simulink model "ee464_hw1_kaantutek_ESR"  (R2022a)
settings: Solver=VariableStepAuto  StartTime=0.0  StopTime=0.5  RelTol=1e-3
libraries: spsGroundLib x14, spsSeriesRLCBranchLib x13, spsCurrentMeasurementLib x7, spsVoltageMeasurementLib x5, spsDCVoltageSourceLib x3, spsDiodeLib x3, spsMosfetLib x3, spsIdealSwitchLib x1, spspowerguiLib x1
settings Model: Creator=mluser  LastModifiedBy=mluser

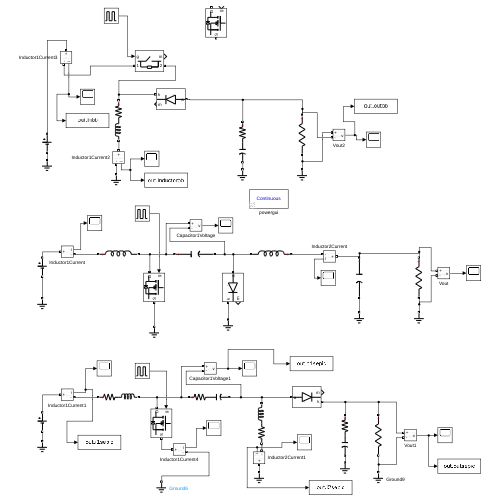
[thumbnail: Simulink's stored preview of the top-level diagram]
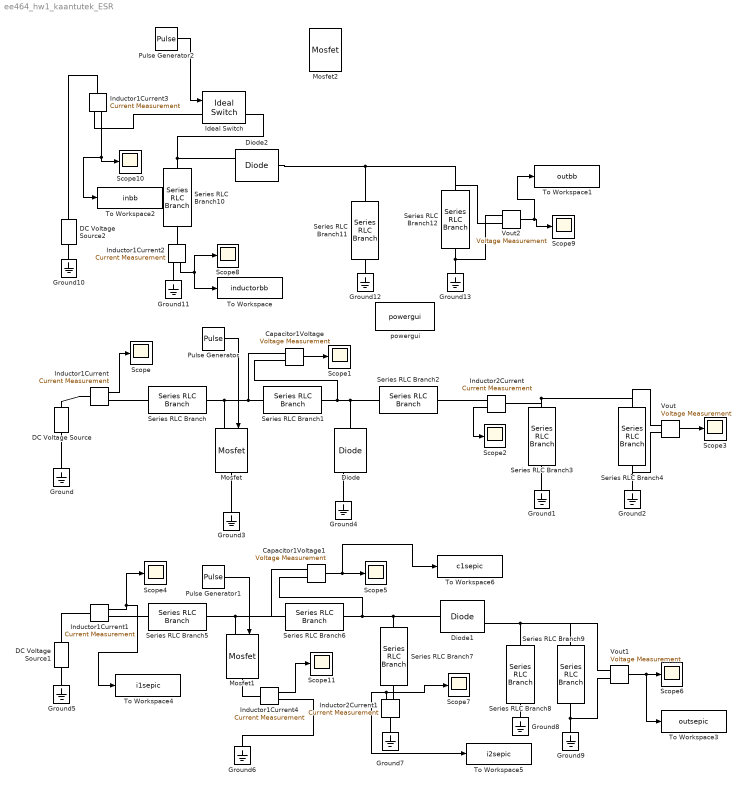
== system ee464_hw1_kaantutek_ESR ==
  Capacitor1Voltage : spsVoltageMeasurementLib/Voltage Measurement  PhasorSimulation=off  OutputType=Complex  PSBequivalent=0
  Capacitor1Voltage1 : spsVoltageMeasurementLib/Voltage Measurement  PhasorSimulation=off  OutputType=Complex  PSBequivalent=0
  DC Voltage Source : spsDCVoltageSourceLib/DC Voltage Source  Amplitude=16  Measurements=None
  DC Voltage Source1 : spsDCVoltageSourceLib/DC Voltage Source  Amplitude=16  Measurements=None
  DC Voltage Source2 : spsDCVoltageSourceLib/DC Voltage Source  Amplitude=16  Measurements=None
  Diode : spsDiodeLib/Diode  Ron=1e-3  Lon=0  Vf=0  IC=0  UseSnubber=0  Rs=0  Cs=0  Measurements=on
  Diode1 : spsDiodeLib/Diode  Ron=1e-3  Lon=0  Vf=0  IC=0  UseSnubber=0  Rs=0  Cs=0  Measurements=on
  Diode2 : spsDiodeLib/Diode  Ron=1e-3  Lon=0  Vf=0  IC=0  UseSnubber=0  Rs=0  Cs=0  Measurements=on
  Ground{,1..13} (14 alike) : spsGroundLib/Ground  LConnTagsString=a
  Ideal Switch : spsIdealSwitchLib/Ideal Switch  Ron=0.001  Lon=0  IC=0  Rs=1e5  Cs=inf  Measurements=on
  Inductor1Current{,1..4} (5 alike) : spsCurrentMeasurementLib/Current Measurement  PhasorSimulation=off  OutputType=Complex  PSBequivalent=0
  Inductor2Current : spsCurrentMeasurementLib/Current Measurement  PhasorSimulation=off  OutputType=Complex  PSBequivalent=0
  Inductor2Current1 : spsCurrentMeasurementLib/Current Measurement  PhasorSimulation=off  OutputType=Complex  PSBequivalent=0
  Mosfet : spsMosfetLib/Mosfet  Ron=1e-6  Lon=0  Rd=1e-6  Vfd=0  IC=0  Rs=1e9  Cs=inf  Measurements=off
  Mosfet1 : spsMosfetLib/Mosfet  Ron=1e-6  Lon=0  Rd=1e-6  Vfd=0  IC=0  Rs=1e9  Cs=inf  Measurements=off
  Mosfet2 : spsMosfetLib/Mosfet  Ron=1e-6  Lon=0  Rd=1e-6  Vfd=0  IC=0  Rs=1e9  Cs=inf  Measurements=off
  Pulse Generator : DiscretePulseGenerator  PulseType=Time based  Amplitude=5  Period=2e-5  PulseWidth=42.857
  Pulse Generator1 : DiscretePulseGenerator  PulseType=Time based  Amplitude=5  Period=2e-5  PulseWidth=42.857
  Pulse Generator2 : DiscretePulseGenerator  PulseType=Time based  Amplitude=5  Period=2e-5  PulseWidth=42.857
  Scope{,1..11} (12 alike) : Scope
  Series RLC Branch : spsSeriesRLCBranchLib/Series RLC Branch  LConnTagsString=__new0  RConnTagsString=__new0  BranchType=L  Resistance=1  Inductance=0.914e-3  SetiL0=off  InitialCurrent=0  Capacitance=1e-6  Setx0=off  InitialVoltage=0  Measurements=None
  Series RLC Branch1 : spsSeriesRLCBranchLib/Series RLC Branch  LConnTagsString=__new0  RConnTagsString=__new0  BranchType=C  Resistance=1  Inductance=1e-3  SetiL0=off  InitialCurrent=0  Capacitance=12.45e-6  Setx0=off  InitialVoltage=0  Measurements=None
  Series RLC Branch10 : spsSeriesRLCBranchLib/Series RLC Branch  LConnTagsString=__new0  RConnTagsString=__new0  BranchType=RL  Resistance=0.048  Inductance=0.470e-3  SetiL0=off  InitialCurrent=0  Capacitance=1e-6  Setx0=off  InitialVoltage=0  Measurements=None
  Series RLC Branch11 : spsSeriesRLCBranchLib/Series RLC Branch  LConnTagsString=__new0  RConnTagsString=__new0  BranchType=RC  Resistance=0.0031  Inductance=1e-3  SetiL0=off  InitialCurrent=0  Capacitance=75e-6  Setx0=off  InitialVoltage=0  Measurements=None
  Series RLC Branch12 : spsSeriesRLCBranchLib/Series RLC Branch  LConnTagsString=__new0  RConnTagsString=__new0  BranchType=R  Resistance=6  Inductance=0  SetiL0=off  InitialCurrent=0  Capacitance=0  Setx0=off  InitialVoltage=0  Measurements=None
  Series RLC Branch2 : spsSeriesRLCBranchLib/Series RLC Branch  LConnTagsString=__new0  RConnTagsString=__new0  BranchType=L  Resistance=1  Inductance=0.686e-3  SetiL0=off  InitialCurrent=0  Capacitance=1e-6  Setx0=off  InitialVoltage=0  Measurements=None
  Series RLC Branch3 : spsSeriesRLCBranchLib/Series RLC Branch  LConnTagsString=__new0  RConnTagsString=__new0  BranchType=C  Resistance=1  Inductance=1e-3  SetiL0=off  InitialCurrent=0  Capacitance=6.12e-6  Setx0=off  InitialVoltage=0  Measurements=None
  Series RLC Branch4 : spsSeriesRLCBranchLib/Series RLC Branch  LConnTagsString=__new0  RConnTagsString=__new0  BranchType=R  Resistance=6  Inductance=0  SetiL0=off  InitialCurrent=0  Capacitance=0  Setx0=off  InitialVoltage=0  Measurements=None
  Series RLC Branch5 : spsSeriesRLCBranchLib/Series RLC Branch  LConnTagsString=__new0  RConnTagsString=__new0  BranchType=RL  Resistance=2.44  Inductance=0.960e-3  SetiL0=off  InitialCurrent=0  Capacitance=1e-6  Setx0=off  InitialVoltage=0  Measurements=None
  Series RLC Branch6 : spsSeriesRLCBranchLib/Series RLC Branch  LConnTagsString=__new0  RConnTagsString=__new0  BranchType=RC  Resistance=10.6e-3  Inductance=1e-3  SetiL0=off  InitialCurrent=0  Capacitance=11e-6  Setx0=off  InitialVoltage=0  Measurements=None
  Series RLC Branch7 : spsSeriesRLCBranchLib/Series RLC Branch  LConnTagsString=__new0  RConnTagsString=__new0  BranchType=RL  Resistance=1.6  Inductance=0.68e-3  SetiL0=off  InitialCurrent=0  Capacitance=1e-6  Setx0=off  InitialVoltage=0  Measurements=None
  Series RLC Branch8 : spsSeriesRLCBranchLib/Series RLC Branch  LConnTagsString=__new0  RConnTagsString=__new0  BranchType=RC  Resistance=5.2e-3  Inductance=1e-3  SetiL0=off  InitialCurrent=0  Capacitance=95e-6  Setx0=off  InitialVoltage=0  Measurements=None
  Series RLC Branch9 : spsSeriesRLCBranchLib/Series RLC Branch  LConnTagsString=__new0  RConnTagsString=__new0  BranchType=R  Resistance=6  Inductance=0  SetiL0=off  InitialCurrent=0  Capacitance=0  Setx0=off  InitialVoltage=0  Measurements=None
  To Workspace : ToWorkspace  VariableName=inductorbb  SaveFormat=Timeseries  SampleTime=-1
  To Workspace1 : ToWorkspace  VariableName=outbb  SaveFormat=Timeseries  SampleTime=-1
  To Workspace2 : ToWorkspace  VariableName=inbb  SaveFormat=Timeseries  SampleTime=-1
  To Workspace3 : ToWorkspace  VariableName=outsepic  SaveFormat=Timeseries  SampleTime=-1
  To Workspace4 : ToWorkspace  VariableName=i1sepic  SaveFormat=Timeseries  SampleTime=-1
  To Workspace5 : ToWorkspace  VariableName=i2sepic  SaveFormat=Timeseries  SampleTime=-1
  To Workspace6 : ToWorkspace  VariableName=c1sepic  SaveFormat=Timeseries  SampleTime=-1
  Vout : spsVoltageMeasurementLib/Voltage Measurement  PhasorSimulation=off  OutputType=Complex  PSBequivalent=0
  Vout1 : spsVoltageMeasurementLib/Voltage Measurement  PhasorSimulation=off  OutputType=Complex  PSBequivalent=0
  Vout2 : spsVoltageMeasurementLib/Voltage Measurement  PhasorSimulation=off  OutputType=Complex  PSBequivalent=0
  powergui : spspowerguiLib/powergui  Priority=1  SimulationMode=Continuous  SampleTime=1e-5  frequency=60  Iterations=50  frequencyindice=0  Pbase=100e6  ErrMax=1e-4  UnitsV=kV  UnitsW=MW  buscounter=0  FunctionMessages=off  echomessages=off  EnableUseOfTLC=off  CurrentSourceSwitches=off  DisableSnubberDevices=off  DisableRonSwitches=off  DisableVfSwitches=off  DisplayEquations=off  AutomaticDiscreteSolvers=off  SolverType=Tustin/Backward Euler (TBE)  Interpol=off  ExternalGateDelay=off  methode=off  Ts=100  x0status=blocks  SPID=on  SwTol=0  HookPort=off  NonlinearTolerance=1e-4  nMaxIteration=100  ContinueOnMaxIteration=off  RestoreLinks=warning  ResistiveCurrentMeasurement=off  Frange=[0:2:500]  Ylog=off  Xlog=on  ShowGrid=off  save=off  variable=ZData  structure=0  ZoomFFT=off  StartTime=0.0  cycles=1  DisplayStyle=1  fundamental=60  FreqAxis=off  MaxFrequency=1000  frequencyindicesteady=1  RmsSteady=1  display=off
  wires:
  Pulse Generator/1 -> Mosfet/1
  Inductor1Current/1 -> Scope/1
  Capacitor1Voltage/1 -> Scope1/1
  Inductor2Current/1 -> Scope2/1
  Vout/1 -> Scope3/1
  Pulse Generator1/1 -> Mosfet1/1
  Inductor1Current1/1 -> To Workspace4/1, Scope4/1
  Capacitor1Voltage1/1 -> To Workspace6/1, Scope5/1
  Vout1/1 -> To Workspace3/1, Scope6/1
  Inductor2Current1/1 -> Scope7/1, To Workspace5/1
  Pulse Generator2/1 -> Ideal Switch/1
  Inductor1Current2/1 -> Scope8/1, To Workspace/1
  Vout2/1 -> To Workspace1/1, Scope9/1
  Inductor1Current3/1 -> To Workspace2/1, Scope10/1
  Inductor1Current4/1 -> Scope11/1
  connections:
  DC Voltage Source/LConn1 -- Ground/LConn1
  Series RLC Branch/RConn1 -- Mosfet/LConn1 -- Capacitor1Voltage/LConn1 -- Series RLC Branch1/LConn1
  Series RLC Branch2/RConn1 -- Diode/LConn1 -- Capacitor1Voltage/LConn2 -- Series RLC Branch1/RConn1
  Ground1/LConn1 -- Series RLC Branch3/RConn1
  Ground2/LConn1 -- Vout/LConn2 -- Series RLC Branch4/RConn1
  Ground4/LConn1 -- Diode/RConn1
  Vout/LConn1 -- Series RLC Branch4/LConn1 -- Inductor2Current/LConn1 -- Series RLC Branch3/LConn1
  Inductor1Current/LConn1 -- DC Voltage Source/RConn1
  Inductor1Current/RConn1 -- Series RLC Branch/LConn1
  Inductor2Current/RConn1 -- Series RLC Branch2/LConn1
  Ground3/LConn1 -- Mosfet/RConn1
  Ground5/LConn1 -- DC Voltage Source1/LConn1
  Mosfet1/LConn1 -- Capacitor1Voltage1/LConn1 -- Series RLC Branch6/LConn1 -- Series RLC Branch5/RConn1
  Series RLC Branch5/LConn1 -- Inductor1Current1/RConn1
  Inductor1Current1/LConn1 -- DC Voltage Source1/RConn1
  Series RLC Branch7/RConn1 -- Capacitor1Voltage1/LConn2 -- Series RLC Branch6/RConn1 -- Diode1/LConn1
  Ground7/LConn1 -- Inductor2Current1/LConn1
  Inductor2Current1/RConn1 -- Series RLC Branch7/LConn1
  Diode1/RConn1 -- Vout1/LConn1 -- Series RLC Branch9/LConn1 -- Series RLC Branch8/LConn1
  Ground8/LConn1 -- Series RLC Branch8/RConn1
  Ground9/LConn1 -- Vout1/LConn2 -- Series RLC Branch9/RConn1
  DC Voltage Source2/LConn1 -- Ground10/LConn1
  Diode2/RConn1 -- Ideal Switch/RConn1 -- Series RLC Branch10/LConn1
  Series RLC Branch10/RConn1 -- Inductor1Current2/LConn1
  Ground11/LConn1 -- Inductor1Current2/RConn1
  Ground12/LConn1 -- Series RLC Branch11/RConn1
  Series RLC Branch12/RConn1 -- Vout2/LConn1 -- Ground13/LConn1
  DC Voltage Source2/RConn1 -- Inductor1Current3/LConn1
  Inductor1Current3/RConn1 -- Ideal Switch/LConn1
  Vout2/LConn2 -- Series RLC Branch12/LConn1 -- Diode2/LConn1 -- Series RLC Branch11/LConn1
  Inductor1Current4/LConn1 -- Mosfet1/RConn1
  Inductor1Current4/RConn1 -- Ground6/LConn1
